simulink model "steady_state_error_type_1_R2017a"  (Simulink 8.9)
settings: Solver=VariableStepAuto  StartTime=0.0  StopTime=100  RelTol=1e-3
model workspace (MAT data in the model file):
  A = Simulink.Parameter
  A.Value = 1
  A.DataType = 'auto'
  A.DocUnits = 'm^2'
  A.Dimensions = [1 1]
  h0 = Simulink.Parameter
  h0.Value = 0
  h0.DataType = 'auto'
  h0.DocUnits = 'm'
  h0.Dimensions = [1 1]
  k1 = Simulink.Parameter
  k1.Value = 10
  k1.DataType = 'auto'
  k1.DocUnits = 'm^2/s'
  k1.Dimensions = [1 1]
  qin = Simulink.Parameter
  qin.Value = 0.4
  qin.DataType = 'auto'
  qin.DocUnits = 'm^3/s'
  qin.Dimensions = [1 1]
settings Model: Creator=waleed.elbadry  LastModifiedBy=waleed.elbadry  OrderedModelArguments=off
settings DataIOCC: LimitDataPoints=off  SaveFormat=Dataset  SignalLoggingSaveFormat=Dataset
settings OptimizationCC: LifeSpan=auto
settings DebuggingCC: UnderspecifiedInitializationDetection=Simplified  MergeDetectMultiDrivingBlocksExec=error  FcnCallInpInsideContextMsg=error  StateNameClashWarn=none  SFUnexpectedBacktrackingDiag=error  SFNoUnconditionalDefaultTransitionDiag=error  SFExecutionAtInitializationDiag=warning
settings HardwareCC: ProdBitPerPointer=64  ProdBitPerSizeT=64  ProdBitPerPtrDiffT=64  ProdLargestAtomicFloat=Float  ProdIntDivRoundTo=Zero  ProdEndianess=LittleEndian  ProdWordSize=64  ProdHWDeviceType=Intel->x86-64 (Windows64)
settings ModelReferenceCC: PropagateSignalLabelsOutOfModel=on
settings SFSimCC: SimUseLocalCustomCode=on
settings RTWCC: RTWUseLocalCustomCode=on
settings GRTTargetCC: TargetLangStandard=C99 (ISO)  GeneratePreprocessorConditionals=Use local settings  CombineOutputUpdateFcns=on  GRTInterface=off
settings ConfigComp: CovMetricSettings=dwe  CovHtmlReporting=off  CovSaveCumulativeToWorkspaceVar=off  CovSaveSingleToWorkspaceVar=off  CovExternalEMLEnable=on

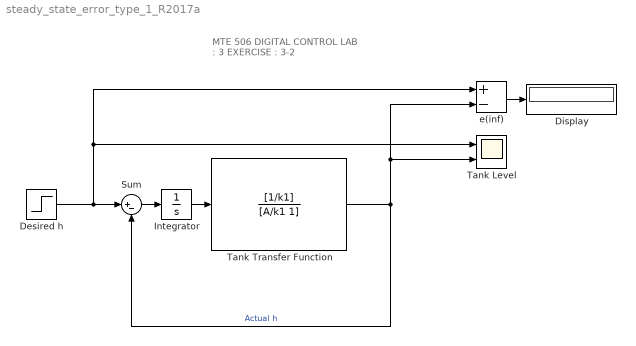
== system steady_state_error_type_1_R2017a ==
  note: MTE 506 DIGITAL CONTROL
      | LAB : 3
      | EXERCISE : 3-2
  Desired h : Step  Time=0  After=4  SampleTime=0
  Display : Display
      settings: Decimation=2
  Integrator : Integrator
  Sum : Sum  Inputs=|+-
  Tank Level : Scope  NumInputPorts=2
  Tank Transfer Function : TransferFcn  Numerator=[1/k1]  Denominator=[A/k1 1]
  e(inf) : Sum  Inputs=+-
  wires:
  Tank Transfer Function/1 -> e(inf)/2, Tank Level/2, Sum/2  "Actual h"
  Desired h/1 -> e(inf)/1, Tank Level/1, Sum/1
  e(inf)/1 -> Display/1
  Sum/1 -> Integrator/1
  Integrator/1 -> Tank Transfer Function/1
